simulink model "Symulacja_z_regulatorem_Simulink"  (Simulink 8.7)
settings: Solver=ode3  StartTime=0.0  StopTime=1000  FixedStep=1  RelTol=1e-3
values from neighbouring files (symbols this model uses):
  k = 16.413    [okreslanie_modelu_obiektu.m]
  offset = Wyniki(1,2)    [okreslanie_modelu_obiektu.m]
  T = 237.67    [okreslanie_modelu_obiektu.m]
  tau = 6.302    [okreslanie_modelu_obiektu.m]
libraries: simulink x1
settings Model: Creator=agnpi  LastModifiedBy=agnpi
settings DataIOCC: LimitDataPoints=off  SaveFormat=Dataset
settings DebuggingCC: UnderspecifiedInitializationDetection=Simplified  MergeDetectMultiDrivingBlocksExec=error
settings HardwareCC: ProdBitPerPointer=64  ProdLargestAtomicFloat=Float  ProdIntDivRoundTo=Zero  ProdEndianess=LittleEndian  ProdWordSize=64  ProdHWDeviceType=Intel->x86-64 (Windows64)
settings ModelReferenceCC: PropagateSignalLabelsOutOfModel=on
settings ConfigComp: CovModelRefEnable=off

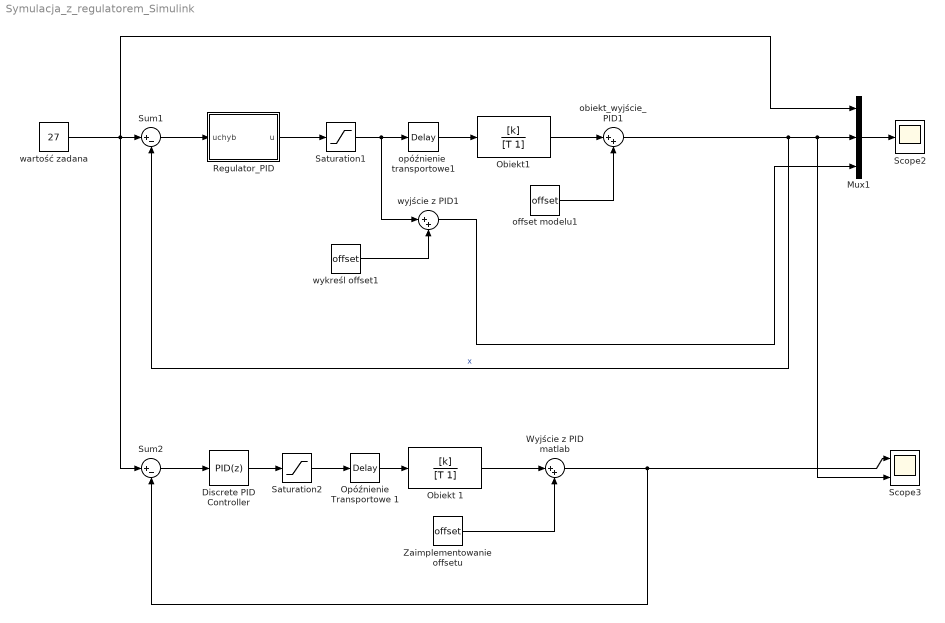
== system Symulacja_z_regulatorem_Simulink ==
  Discrete PID Controller : simulink/Continuous/PID Controller  Controller=PID  TimeDomain=Discrete-time  SampleTime=1  IntegratorMethod=Trapezoidal  FilterMethod=Forward Euler  Form=Parallel  UseFilter=off  ControllerParametersSource=internal  P=0.52  I=0.003  D=0.257  N=100  InitialConditionSource=internal  InitialConditionForIntegrator=0  InitialConditionForFilter=0  ExternalReset=none  LimitOutput=on  UpperSaturationLimit=1  LowerSaturationLimit=0  LinearizeAsGain=off  AntiWindupMode=none  Kb=1  TrackingMode=off  Kt=1  PParamMin=[]  PParamMax=[]  IParamMin=[]  IParamMax=[]  DParamMin=[]  DParamMax=[]  NParamMin=[]  NParamMax=[]  KbParamMin=[]  KbParamMax=[]  KtParamMin=[]  KtParamMax=[]  POutMin=[]  POutMax=[]  IOutMin=[]  IOutMax=[]  DOutMin=[]  DOutMax=[]  NOutMin=[]  NOutMax=[]  KbOutMin=[]  KbOutMax=[]  KtOutMin=[]  KtOutMax=[]  IntegratorOutMin=[]  IntegratorOutMax=[]  FilterOutMin=[]  FilterOutMax=[]  SumOutMin=[]  SumOutMax=[]  SumI1OutMin=[]  SumI1OutMax=[]  SumI2OutMin=[]  SumI2OutMax=[]  SumI3OutMin=[]  SumI3OutMax=[]  SumDOutMin=[]  SumDOutMax=[]  SaturationOutMin=[]  SaturationOutMax=[]  IntegratorContinuousStateAttributes=''  IntegratorStateMustResolveToSignalObject=off  IntegratorRTWStateStorageClass=Auto  FilterContinuousStateAttributes=''  FilterStateMustResolveToSignalObject=off  FilterRTWStateStorageClass=Auto  DifferentiatorICPrevScaledInput=0  DifferentiatorOutMin=[]  DifferentiatorOutMax=[]
  Mux1 : Mux  Inputs=3
  Obiekt 1 : TransferFcn  Numerator=[k]  Denominator=[T 1]
  Obiekt1 : TransferFcn  Numerator=[k]  Denominator=[T 1]
  "Opóźnienie Transportowe 1 " : TransportDelay  DelayTime=tau
  Regulator_PID : MATLAB Function  TreatAsAtomicUnit=on
  Saturation1 : Saturate  UpperLimit=1  LowerLimit=0
  Saturation2 : Saturate  UpperLimit=1  LowerLimit=0
  Scope2 : Scope
  Scope3 : Scope  NumInputPorts=2
  Sum1 : Sum  Inputs=|+-
  Sum2 : Sum  Inputs=|+-
  Wyjście z PID matlab : Sum  Inputs=|++
  "Zaimplementowanie offsetu " : Constant  Value=offset  SampleTime=-1
  obiekt_wyjście_PID1 : Sum  Inputs=|++
  offset modelu1 : Constant  Value=offset  SampleTime=-1
  opóźnienie  transportowe1 : TransportDelay  DelayTime=tau
  wartość zadana : Constant  Value=27
  wyjście z PID1 : Sum  Inputs=|++
  wykreśl offset1 : Constant  Value=offset
  wires:
  wartość zadana/1 -> Sum2/1, Mux1/1, Sum1/1
  obiekt_wyjście_PID1/1 -> Scope3/2, Mux1/2, Sum1/2  "x"
  Sum1/1 -> Regulator_PID/1(uchyb)
  Regulator_PID/1(u) -> Saturation1/1
  opóźnienie  transportowe1/1 -> Obiekt1/1
  offset modelu1/1 -> obiekt_wyjście_PID1/2
  Obiekt1/1 -> obiekt_wyjście_PID1/1
  Saturation1/1 -> wyjście z PID1/1, opóźnienie  transportowe1/1
  wykreśl offset1/1 -> wyjście z PID1/2
  wyjście z PID1/1 -> Mux1/3
  Mux1/1 -> Scope2/1
  Obiekt 1/1 -> Wyjście z PID matlab/1
  "Zaimplementowanie offsetu "/1 -> Wyjście z PID matlab/2
  Saturation2/1 -> "Opóźnienie Transportowe 1 "/1
  "Opóźnienie Transportowe 1 "/1 -> Obiekt 1/1
  Discrete PID Controller/1 -> Saturation2/1
  Sum2/1 -> Discrete PID Controller/1
  Wyjście z PID matlab/1 -> Scope3/1, Sum2/2

== matlab function Regulator_PID ==
  data: uchyb input double; u output double
function u = Regulator_PID(uchyb)

% Deklaracja ststycznych wartości
persistent poprzedni_uchyb;
if isempty(poprzedni_uchyb)
    poprzedni_uchyb = 0;
end

persistent poprzednia_calka;
if isempty(poprzednia_calka)
    poprzednia_calka = 0;
end

% Stałe wartości 
% !!!!(TU PODAJEMY NASZE WARTOŚĆI PID z Tunera z bloku PID Discrete)!!!!:
dt = 1;
Kp = 0.52;
Ki = 0.003;
Kd = 0.257;
% N = 100;

% Część proporcjonalna:
P = Kp*uchyb;

% Część całkująca:
calka = poprzednia_calka + (uchyb+poprzedni_uchyb) ; % integrator bez anti-windup
poprzednia_calka = calka;
I = Ki*calka*(dt/2);

% Człon rózniczkujący:
rozniczka = (uchyb - poprzedni_uchyb)/dt; % numeryczna rózniczka bez filtra
D = Kd*rozniczka;


% Suma wszystkich części:
u = P  + I + D; % bez saturacji
